simulink model "CSE1_DP"  (R2014a)
settings: Solver=ode4  StartTime=0.0  StopTime=time  FixedStep=h  RelTol=1e-3
values from neighbouring files (symbols this model uses):
  head_pitch = 0    [run_file.m]
  Head_roll = 0    [run_file.m]
  head_yaw = 0    [run_file.m]
  K_2_psi = 30    [run_file.m]
  K_2_x = 30    [run_file.m]
  K_2_y = 30    [run_file.m]
  K_3_psi = 2    [run_file.m]
  K_3_x = 2    [run_file.m]
  K_3_y = 2    [run_file.m]
  K_4_psi = 2    [run_file.m]
  K_4_x = 2    [run_file.m]
  K_4_y = 2    [run_file.m]
  K_d_psi = 8    [run_file.m]
  K_d_x = 8    [run_file.m]
  K_d_y = 8    [run_file.m]
  K_ff_r = 0    [run_file.m]
  K_ff_r_dot = 0    [run_file.m]
  K_ff_u = 0    [run_file.m]
  K_ff_u_dot = 0    [run_file.m]
  K_ff_v = 0    [run_file.m]
  K_ff_v_dot = 0    [run_file.m]
  K_i_psi = 0    [run_file.m]
  K_i_x = 0    [run_file.m]
  K_i_y = 0    [run_file.m]
  K_p_psi = 3    [run_file.m]
  K_p_x = 3    [run_file.m]
  K_p_y = 3    [run_file.m]
  K_r = 0.5    [run_file.m]
  K_u = 1    [run_file.m]
  K_v = 0.5    [run_file.m]
  L = 1    [plot_script.m]    (also in run_file.m = diag([1 1 1]))
  M = [m_11 0    0 ... (first row only)    [run_file.m]
  psi_0 = 1    [run_file.m]
  psi_ref = ref(4,:)    [plot_script.m]    (also in run_file.m = 3.14159265359)
  v_max = [0.3 0.1 1]    [run_file.m]
  w_d_psi = 2    [run_file.m]
  w_d_psi_2 = 2    [run_file.m]
  w_d_x = 1    [run_file.m]
  w_d_x_2 = 1    [run_file.m]
  w_d_y = 1    [run_file.m]
  w_d_y_2 = 1    [run_file.m]
  x_0 = 5    [run_file.m]
  x_ref = ref(2,:)    [plot_script.m]    (also in run_file.m = 4)
  y_0 = 5    [run_file.m]
  y_ref = ref(3,:)    [plot_script.m]    (also in run_file.m = 3)
  zeta_psi = 1    [run_file.m]
  zeta_psi_2 = 1    [run_file.m]
  zeta_x = 1    [run_file.m]
  zeta_x_2 = 1    [run_file.m]
  zeta_y = 1    [run_file.m]
  zeta_y_2 = 1    [run_file.m]
libraries: marine_gnc x15, simulink x2
(part 1 of 2)
settings Model: Creator=Eirik Valle  LastModifiedBy=mclab

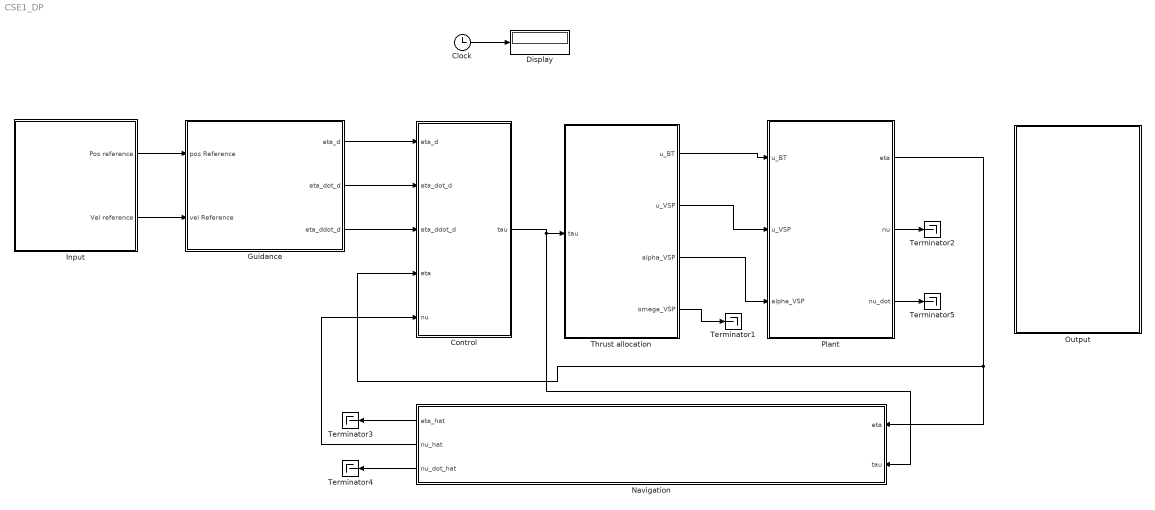
== system CSE1_DP ==
  Clock : Clock
  Control : Subsystem
  Display : Display
  Guidance : Subsystem
  Input : Subsystem
  "Navigation " : Subsystem
  Output : Subsystem
  Plant : Subsystem
  Terminator{1..5} (5 alike) : Terminator
  Thrust allocation : Subsystem
  wires:
  Control/1(tau) -> "Navigation "/2(tau), Thrust allocation/1(tau)
  Plant/1(eta) -> Control/4(eta), "Navigation "/1(eta)
  Input/1(Pos reference) -> Guidance/1("pos Reference ")
  Guidance/1(eta_d) -> Control/1(eta_d)
  Guidance/3(eta_ddot_d) -> Control/3(eta_ddot_d)
  Guidance/2(eta_dot_d) -> Control/2(eta_dot_d)
  "Navigation "/1(eta_hat) -> Terminator3/1
  "Navigation "/3(nu_dot_hat) -> Terminator4/1
  Plant/3(nu_dot) -> Terminator5/1
  Clock/1 -> Display/1
  "Navigation "/2(nu_hat) -> Control/5(nu)
  Plant/2(nu) -> Terminator2/1
  Thrust allocation/1(u_BT) -> Plant/1(u_BT)
  Thrust allocation/2(u_VSP) -> Plant/2(u_VSP)
  Thrust allocation/3(alpha_VSP) -> Plant/3(alpha_VSP)
  Thrust allocation/4(omega_VSP) -> Terminator1/1
  Input/2(Vel reference) -> Guidance/2("vel Reference ")

== system CSE1_DP/Control ==
  eta_d : Inport
  eta_dot_d : Inport  Port=2
  eta_ddot_d : Inport  Port=3
  eta : Inport  Port=4
  nu : Inport  Port=5
  Adaptive law : Subsystem  Commented=on
  Backstepping : Subsystem  Commented=on
  DP Controller : Subsystem
  MRAC : Subsystem  Commented=on
  Manual Switch : ManualSwitch  Commented=on
  tau : Outport
  tag scope: tau=global
  wires:
  eta_d/1 -> DP Controller/1(eta_d)
  eta/1 -> DP Controller/2(eta)
  nu/1 -> DP Controller/3(nu)
  DP Controller/1(tau) -> tau/1, [tau]
  eta_ddot_d/1 -> DP Controller/5(eta_ddot)
  eta_dot_d/1 -> DP Controller/4(eta_dot_d)
  Adaptive law/1(theta) -> MRAC/7(theta)

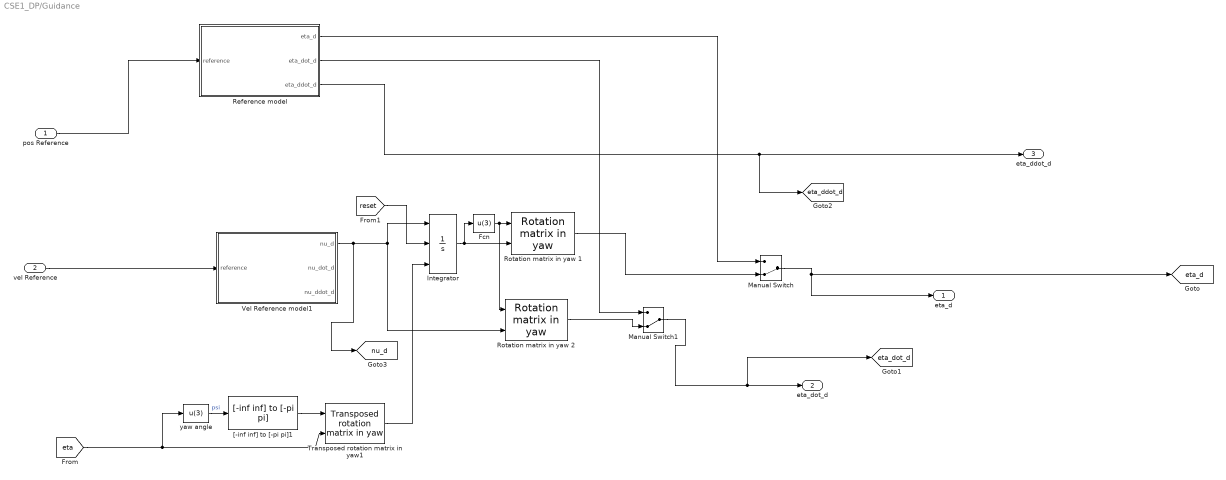
== system CSE1_DP/Guidance ==
  "pos Reference " : Inport
  "vel Reference " : Inport  Port=2
  Fcn : Fcn  Expr=u(3)
  Integrator : Integrator  ExternalReset=either  InitialConditionSource=external
  Manual Switch : ManualSwitch  CurrentSetting=0
  Manual Switch1 : ManualSwitch  CurrentSetting=0
  Reference model : Subsystem
  Rotation matrix in yaw 1 : marine_gnc/Models/ Kinematics/Rotation matrix in yaw 
  Rotation matrix in yaw 2 : marine_gnc/Models/ Kinematics/Rotation matrix in yaw 
  Transposed rotation matrix in yaw1 : marine_gnc/Models/ Kinematics/Transposed rotation  matrix in yaw
  Vel Reference model1 : Subsystem
  "[-inf inf] to [-pi pi]1" : marine_gnc/Utilities/Math Operations/[-inf inf] to [-pi pi]
  yaw angle : Fcn  Expr=u(3)
  eta_d : Outport
  eta_dot_d : Outport  Port=2
  eta_ddot_d : Outport  Port=3
  tag scope: eta_d=global, eta_ddot_d=global, eta_dot_d=global, nu_d=global
  wires:
  Manual Switch/1 -> eta_d/1, [eta_d]
  Manual Switch1/1 -> [eta_dot_d], eta_dot_d/1
  Reference model/3(eta_ddot_d) -> [eta_ddot_d], eta_ddot_d/1
  "pos Reference "/1 -> Reference model/1(reference)
  "vel Reference "/1 -> Vel Reference model1/1(reference)
  Integrator/1 -> Fcn/1, Rotation matrix in yaw 1/2
  Rotation matrix in yaw 1/1 -> Manual Switch/2
  Vel Reference model1/1(nu_d) -> [nu_d], Rotation matrix in yaw 2/2, Integrator/1
  Fcn/1 -> Rotation matrix in yaw 2/1, Rotation matrix in yaw 1/1
  Reference model/1(eta_d) -> Manual Switch/1
  Rotation matrix in yaw 2/1 -> Manual Switch1/2
  Reference model/2(eta_dot_d) -> Manual Switch1/1
  Transposed rotation matrix in yaw1/1 -> Integrator/3
  [reset] -> Integrator/2
  "[-inf inf] to [-pi pi]1"/1 -> Transposed rotation matrix in yaw1/1
  yaw angle/1 -> "[-inf inf] to [-pi pi]1"/1  "psi"
  [eta] -> yaw angle/1, Transposed rotation matrix in yaw1/2

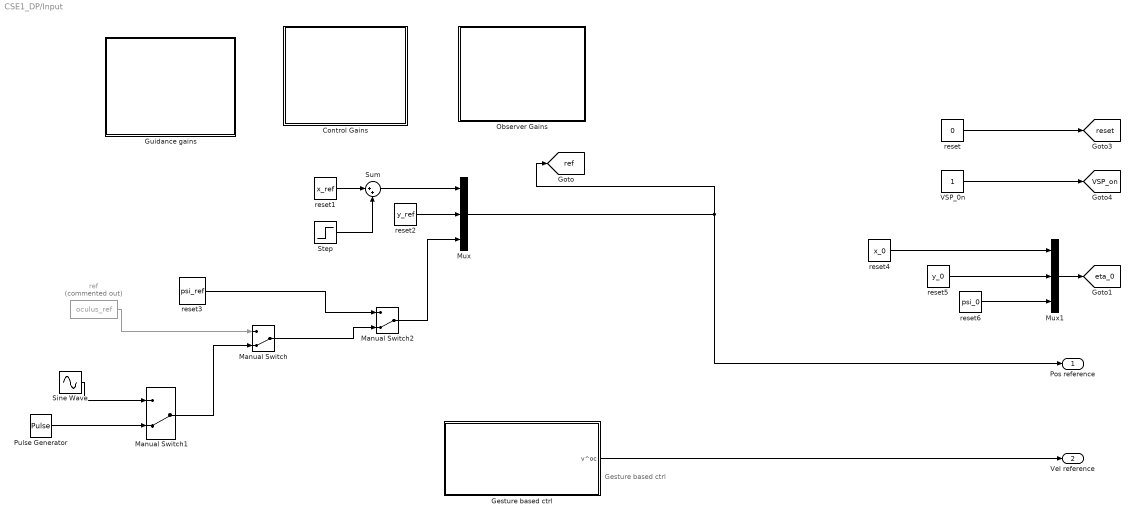
== system CSE1_DP/Input ==
  note: Gesture based ctrl
  Control Gains : Subsystem
  Gesture based ctrl : Subsystem
  Guidance gains : Subsystem
  Manual Switch : ManualSwitch  CurrentSetting=0
  Manual Switch1 : ManualSwitch  CurrentSetting=0
  Manual Switch2 : ManualSwitch  CurrentSetting=0
  Mux : Mux  Inputs=3
  Mux1 : Mux  Inputs=3
  Observer Gains : Subsystem
  Pulse Generator : DiscretePulseGenerator  PulseType=Time based  Amplitude=pi*0.9  Period=30  PulseWidth=50
  Sine Wave : Sin  Amplitude=pi/2  Frequency=0.2  SampleTime=0
  Step : Step  Time=100  After=2  SampleTime=0
  Sum : Sum  Inputs=|++
  VSP_0n : Constant
  ref : FromWorkspace  Commented=on  VariableName=oculus_ref  SampleTime=0
  reset : Constant  Value=0
  reset1 : Constant  Value=x_ref
  reset2 : Constant  Value=y_ref
  reset3 : Constant  Value=psi_ref
  reset4 : Constant  Value=x_0
  reset5 : Constant  Value=y_0
  reset6 : Constant  Value=psi_0
  Pos reference : Outport
  Vel reference : Outport  Port=2
  tag scope: VSP_on=global, eta_0=global, ref=global, reset=global
  wires:
  Mux/1 -> Pos reference/1, [ref]
  reset/1 -> [reset]
  VSP_0n/1 -> [VSP_on]
  reset1/1 -> Sum/1
  reset2/1 -> Mux/2
  reset3/1 -> Manual Switch2/1
  reset4/1 -> Mux1/1
  reset5/1 -> Mux1/2
  reset6/1 -> Mux1/3
  Mux1/1 -> [eta_0]
  ref/1 -> Manual Switch/1
  Manual Switch/1 -> Manual Switch2/2
  Pulse Generator/1 -> Manual Switch1/2
  Sine Wave/1 -> Manual Switch1/1
  Manual Switch1/1 -> Manual Switch/2
  Manual Switch2/1 -> Mux/3
  Sum/1 -> Mux/1
  Step/1 -> Sum/2
  Gesture based ctrl/1("v^oc ") -> Vel reference/1

== system CSE1_DP/Navigation  ==
  eta : Inport
  tau : Inport  Port=2
  Derivative filter : Subsystem
  Manual Switch : ManualSwitch  CurrentSetting=0
  Manual Switch1 : ManualSwitch  CurrentSetting=0
  Nonlinear Passisve Observer : Subsystem
  Terminator : Terminator
  tau_2_tau_actual : Subsystem
  eta_hat : Outport
  nu_hat : Outport  Port=2
  nu_dot_hat : Outport  Port=3
  tag scope: b_hat=global, eta_hat=global, nu_dot_hat=global, nu_hat=global
  wires:
  tau/1 -> Manual Switch/1, tau_2_tau_actual/1(tau)
  Nonlinear Passisve Observer/1(eta_hat) -> [eta_hat], eta_hat/1
  Manual Switch1/1 -> nu_hat/1, [nu_hat]
  Nonlinear Passisve Observer/4(b_hat) -> Terminator/1, [b_hat]
  Nonlinear Passisve Observer/3(nu_dot_hat) -> [nu_dot_hat], nu_dot_hat/1
  Manual Switch/1 -> Nonlinear Passisve Observer/2(tau)
  tau_2_tau_actual/1(tau_actual) -> Manual Switch/2
  eta/1 -> Derivative filter/1(eta), Nonlinear Passisve Observer/1(eta)
  Nonlinear Passisve Observer/2(nu_hat) -> Manual Switch1/1, tau_2_tau_actual/2(nu_hat)
  Derivative filter/1(nu_hat) -> Manual Switch1/2

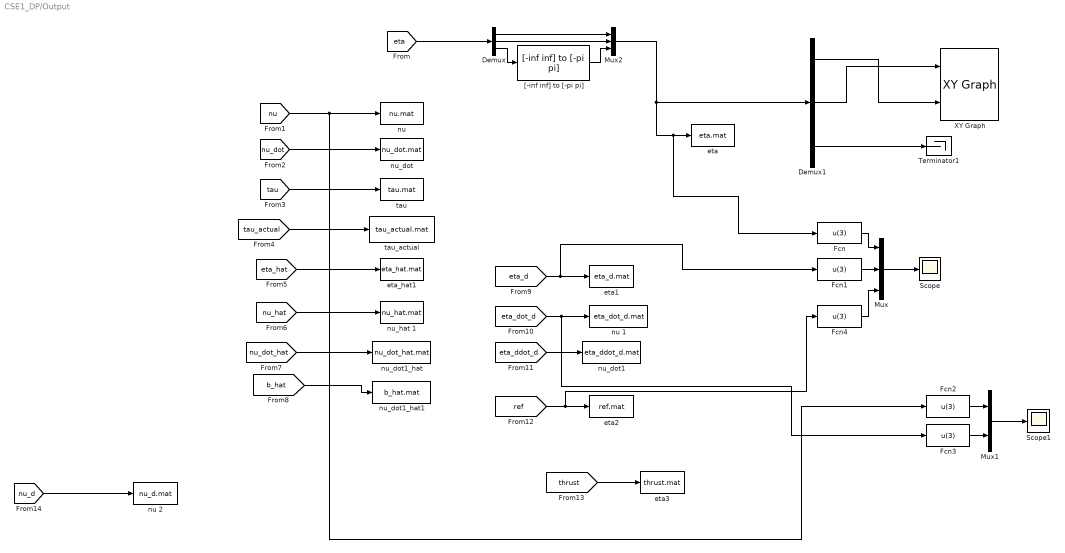
== system CSE1_DP/Output ==
  Demux : Demux  Outputs=3
  Demux1 : Demux  Outputs=3
  Fcn{,1..4} (5 alike) : Fcn  Expr=u(3)
  Mux : Mux  Inputs=3
  Mux1 : Mux  Inputs=2
  Mux2 : Mux  Inputs=3
  Scope : Scope
      settings: YMin=-3.5  YMax=3.5
  Scope1 : Scope
      settings: YMin=-0.1  YMax=0.9
  Terminator1 : Terminator
  XY Graph : simulink/Sinks/XY Graph  xmin=-10  xmax=10  ymin=-10  ymax=10  st=-1
  "[-inf inf] to [-pi pi]" : marine_gnc/Utilities/Math Operations/[-inf inf] to [-pi pi]
  eta : ToFile  Filename=eta.mat  MatrixName=eta
  eta1 : ToFile  Filename=eta_d.mat  MatrixName=eta_d
  eta2 : ToFile  Filename=ref.mat  MatrixName=ref
  eta3 : ToFile  Filename=thrust.mat  MatrixName=thrust
  eta_hat1 : ToFile  Filename=eta_hat.mat  MatrixName=eta_hat
  "nu " : ToFile  Filename=nu.mat  MatrixName=nu
  nu 1 : ToFile  Filename=eta_dot_d.mat  MatrixName=eta_dot_d
  nu 2 : ToFile  Filename=nu_d.mat  MatrixName=nu_d
  nu_dot : ToFile  Filename=nu_dot.mat  MatrixName=nu_dot
  nu_dot1 : ToFile  Filename=eta_ddot_d.mat  MatrixName=eta_ddot_d
  nu_dot1_hat : ToFile  Filename=nu_dot_hat.mat  MatrixName=nu_dot_hat
  nu_dot1_hat1 : ToFile  Filename=b_hat.mat  MatrixName=b_hat
  nu_hat 1 : ToFile  Filename=nu_hat.mat  MatrixName=nu_hat
  tau : ToFile  Filename=tau.mat  MatrixName=tau
  tau_actual : ToFile  Filename=tau_actual.mat  MatrixName=tau_actual
  wires:
  [nu] -> Fcn2/1, "nu "/1
  [nu_dot] -> nu_dot/1
  [tau] -> tau/1
  [tau_actual] -> tau_actual/1
  [eta_hat] -> eta_hat1/1
  [nu_hat] -> nu_hat 1/1
  [nu_dot_hat] -> nu_dot1_hat/1
  [b_hat] -> nu_dot1_hat1/1
  [eta_d] -> Fcn1/1, eta1/1
  [eta_ddot_d] -> nu_dot1/1
  Mux2/1 -> Fcn/1, eta/1, Demux1/1
  Demux1/3 -> Terminator1/1
  Demux1/1 -> XY Graph/2
  Demux1/2 -> XY Graph/1
  [ref] -> Fcn4/1, eta2/1
  [thrust] -> eta3/1
  Mux/1 -> Scope/1
  Fcn/1 -> Mux/1
  Fcn1/1 -> Mux/2
  [eta_dot_d] -> Fcn3/1, nu 1/1
  Mux1/1 -> Scope1/1
  Fcn2/1 -> Mux1/1
  Fcn3/1 -> Mux1/2
  Demux/1 -> Mux2/1
  Demux/2 -> Mux2/2
  "[-inf inf] to [-pi pi]"/1 -> Mux2/3
  Demux/3 -> "[-inf inf] to [-pi pi]"/1
  [eta] -> Demux/1
  Fcn4/1 -> Mux/3
  [nu_d] -> nu 2/1

== system CSE1_DP/Plant ==
  u_BT : Inport
  u_VSP : Inport  Port=2
  alpha_VSP : Inport  Port=3
  CSE1 nonlinear with thruster dynamics : Subsystem
  Terminator : Terminator
  eta : Outport
  nu : Outport  Port=2
  nu_dot : Outport  Port=3
  tag scope: eta=global, nu=global, nu_dot=global, tau_actual=global
  wires:
  CSE1 nonlinear with thruster dynamics/4(nu_dot) -> nu_dot/1, [nu_dot]
  CSE1 nonlinear with thruster dynamics/3(nu) -> [nu], nu/1
  CSE1 nonlinear with thruster dynamics/2(eta) -> eta/1, [eta]
  CSE1 nonlinear with thruster dynamics/1(tau_actual) -> [tau_actual], Terminator/1
  alpha_VSP/1 -> CSE1 nonlinear with thruster dynamics/3(alpha)
  u_VSP/1 -> CSE1 nonlinear with thruster dynamics/2(u_VSP)
  u_BT/1 -> CSE1 nonlinear with thruster dynamics/1(u_bt)

== system CSE1_DP/Thrust allocation ==
  tau : Inport
  linear thrust allocation : Subsystem
  u_BT : Outport
  u_VSP : Outport  Port=2
  alpha_VSP : Outport  Port=3
  omega_VSP : Outport  Port=4
  tag scope: thrust=global
  wires:
  tau/1 -> linear thrust allocation/1(tau)
  linear thrust allocation/5(thrust) -> [thrust]
  linear thrust allocation/1(u_BT) -> u_BT/1
  linear thrust allocation/2(u_VSP) -> u_VSP/1
  linear thrust allocation/3(alpha_VSP) -> alpha_VSP/1
  linear thrust allocation/4(omega_VSP) -> omega_VSP/1

== system CSE1_DP/Control/Adaptive law ==
  a_psi : Inport
  r : Inport  Port=2
  r_d : Inport  Port=3
  Abs : Abs
  Demux : Demux  Outputs=2
  Integrator : Integrator  InitialCondition=[0.01 0.01]
  Matrix Multiply : Product  Multiplication=Matrix(*)
  Mux2 : Mux  Inputs=2
  Product : Product
  Product2 : Product
  Sum : Sum  Inputs=|+-
  theta : Outport
  tag scope: theta_1=global, theta_2=global
  wires:
  Matrix Multiply/1 -> Integrator/1
  Product/1 -> Matrix Multiply/2
  Integrator/1 -> Demux/1, theta/1
  Sum/1 -> Product/2
  Product2/1 -> Mux2/2
  a_psi/1 -> Mux2/1
  r/1 -> Sum/1, Product2/2, Abs/1
  Abs/1 -> Product2/1
  r_d/1 -> Sum/2
  Mux2/1 -> Product/1
  Demux/1 -> [theta_1]
  Demux/2 -> [theta_2]
  [iG5] -> Matrix Multiply/1

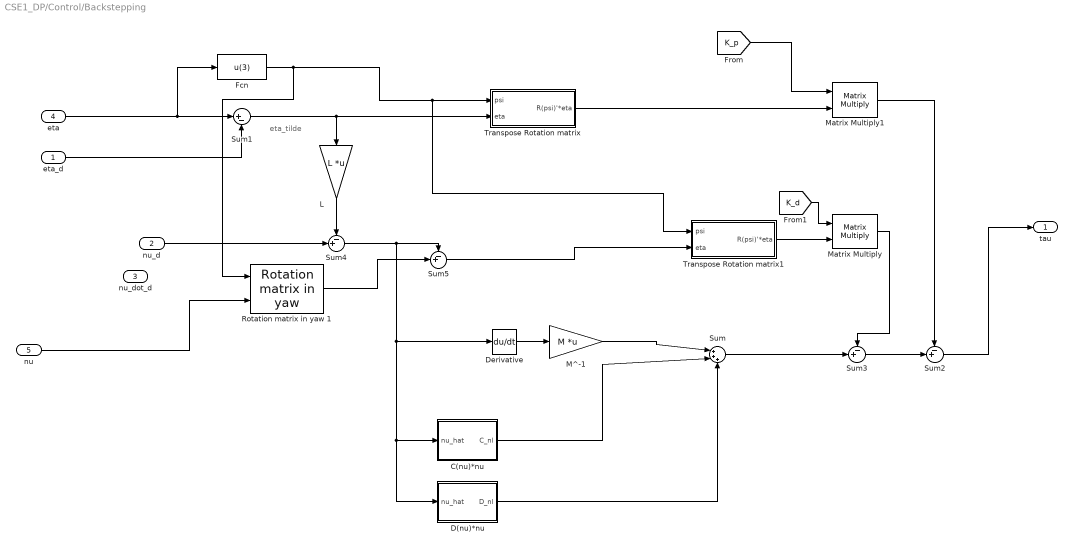
== system CSE1_DP/Control/Backstepping ==
  note: eta_tilde
  eta_d : Inport
  nu_d : Inport  Port=2
  nu_dot_d : Inport  Port=3
  eta : Inport  Port=4
  nu : Inport  Port=5
  C(nu)*nu : MATLAB Function  TreatAsAtomicUnit=on
  D(nu)*nu : MATLAB Function  TreatAsAtomicUnit=on
  Derivative : Derivative
  Fcn : Fcn  Expr=u(3)
  L : Gain  Gain=L  Multiplication=Matrix(K*u)
  M^-1 : Gain  Gain=M  Multiplication=Matrix(K*u)
  Matrix Multiply : Product  Multiplication=Matrix(*)
  Matrix Multiply1 : Product  Multiplication=Matrix(*)
  Rotation matrix in yaw 1 : marine_gnc/Models/ Kinematics/Rotation matrix in yaw 
  Sum : Sum  Inputs=|+++
  Sum1 : Sum  Inputs=|+-
  Sum{2..5} (4 alike) : Sum  Inputs=-+|
  Transpose Rotation matrix : Subsystem
  Transpose Rotation matrix1 : Subsystem
  tau : Outport
  wires:
  nu/1 -> Rotation matrix in yaw 1/2
  Derivative/1 -> M^-1/1
  M^-1/1 -> Sum/1
  C(nu)*nu/1(C_nl) -> Sum/2
  D(nu)*nu/1(D_nl) -> Sum/3
  eta/1 -> Fcn/1, Sum1/1
  eta_d/1 -> Sum1/2
  Sum1/1 -> L/1, Transpose Rotation matrix/2(eta)
  Fcn/1 -> Rotation matrix in yaw 1/1, Transpose Rotation matrix1/1(psi), Transpose Rotation matrix/1(psi)
  Sum/1 -> Sum3/2
  Transpose Rotation matrix/1(R(psi)'*eta) -> Matrix Multiply1/2
  Sum3/1 -> Sum2/2
  nu_d/1 -> Sum4/2
  L/1 -> Sum4/1
  Transpose Rotation matrix1/1(R(psi)'*eta) -> Matrix Multiply/2
  Sum5/1 -> Transpose Rotation matrix1/2(eta)
  Matrix Multiply1/1 -> Sum2/1
  [K_p] -> Matrix Multiply1/1
  [K_d] -> Matrix Multiply/1
  Matrix Multiply/1 -> Sum3/1
  Rotation matrix in yaw 1/1 -> Sum5/2
  Sum2/1 -> tau/1
  Sum4/1 -> Derivative/1, D(nu)*nu/1(nu_hat), C(nu)*nu/1(nu_hat), Sum5/1

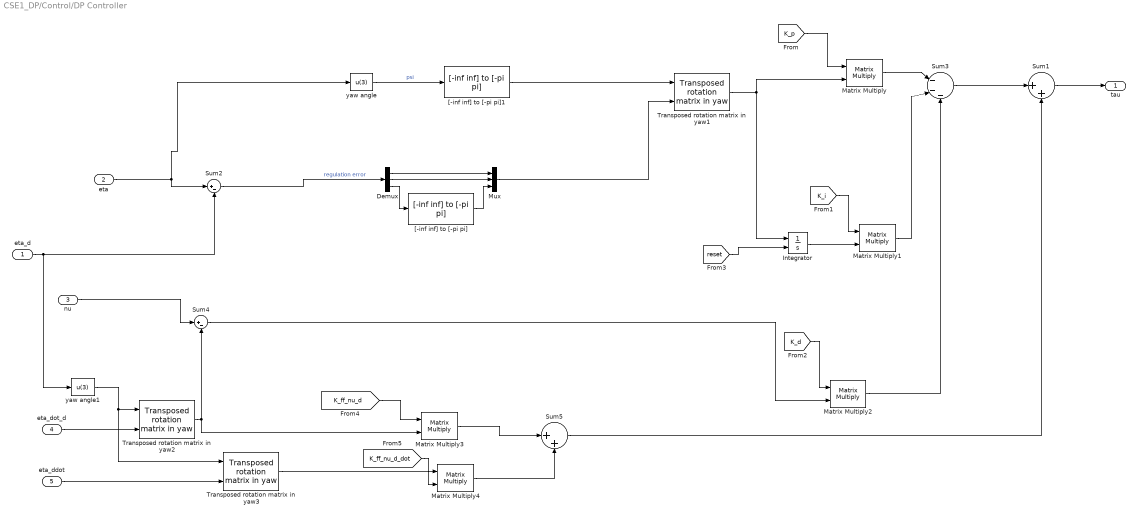
== system CSE1_DP/Control/DP Controller ==
  eta_d : Inport
  eta : Inport  Port=2
  nu : Inport  Port=3
  eta_dot_d : Inport  Port=4
  eta_ddot : Inport  Port=5
  Demux : Demux  Outputs=3
  Integrator : Integrator  ExternalReset=either
  Matrix Multiply{,1..4} (5 alike) : Product  Multiplication=Matrix(*)
  Mux : Mux  Inputs=3
  Sum1 : Sum  Inputs=|++  SaturateOnIntegerOverflow=on  InputSameDT=on  OutDataTypeStr=Inherit: Same as first input
  Sum2 : Sum  Inputs=|+-  SaturateOnIntegerOverflow=on  InputSameDT=on  OutDataTypeStr=Inherit: Same as first input
  Sum3 : Sum  Inputs=|---  SaturateOnIntegerOverflow=on  InputSameDT=on  OutDataTypeStr=Inherit: Same as first input
  Sum4 : Sum  Inputs=|+-  SaturateOnIntegerOverflow=on  InputSameDT=on  OutDataTypeStr=Inherit: Same as first input
  Sum5 : Sum  Inputs=|++  SaturateOnIntegerOverflow=on  InputSameDT=on  OutDataTypeStr=Inherit: Same as first input
  Transposed rotation matrix in yaw1 : marine_gnc/Models/ Kinematics/Transposed rotation  matrix in yaw
  Transposed rotation matrix in yaw2 : marine_gnc/Models/ Kinematics/Transposed rotation  matrix in yaw
  Transposed rotation matrix in yaw3 : marine_gnc/Models/ Kinematics/Transposed rotation  matrix in yaw
  "[-inf inf] to [-pi pi]" : marine_gnc/Utilities/Math Operations/[-inf inf] to [-pi pi]
  "[-inf inf] to [-pi pi]1" : marine_gnc/Utilities/Math Operations/[-inf inf] to [-pi pi]
  yaw angle : Fcn  Expr=u(3)
  yaw angle1 : Fcn  Expr=u(3)
  tau : Outport  InitialOutput=0
  wires:
  "[-inf inf] to [-pi pi]1"/1 -> Transposed rotation matrix in yaw1/1
  yaw angle/1 -> "[-inf inf] to [-pi pi]1"/1  "psi"
  Mux/1 -> Transposed rotation matrix in yaw1/2
  Demux/1 -> Mux/1
  Demux/2 -> Mux/2
  "[-inf inf] to [-pi pi]"/1 -> Mux/3
  Sum2/1 -> Demux/1  "regulation error"
  Demux/3 -> "[-inf inf] to [-pi pi]"/1
  Sum3/1 -> Sum1/1
  eta/1 -> Sum2/1, yaw angle/1
  nu/1 -> Sum4/1
  Matrix Multiply2/1 -> Sum3/3
  Integrator/1 -> Matrix Multiply1/2
  Matrix Multiply/1 -> Sum3/1
  Matrix Multiply1/1 -> Sum3/2
  Transposed rotation matrix in yaw1/1 -> Integrator/1, Matrix Multiply/2
  eta_d/1 -> yaw angle1/1, Sum2/2
  [reset] -> Integrator/2
  [K_p] -> Matrix Multiply/1
  [K_i] -> Matrix Multiply1/1
  [K_d] -> Matrix Multiply2/1
  eta_dot_d/1 -> Transposed rotation matrix in yaw2/2
  Transposed rotation matrix in yaw2/1 -> Sum4/2, Matrix Multiply3/2
  Sum4/1 -> Matrix Multiply2/2
  yaw angle1/1 -> Transposed rotation matrix in yaw3/1, Transposed rotation matrix in yaw2/1
  Sum1/1 -> tau/1
  eta_ddot/1 -> Transposed rotation matrix in yaw3/2
  Transposed rotation matrix in yaw3/1 -> Matrix Multiply4/2
  Matrix Multiply3/1 -> Sum5/1
  Sum5/1 -> Sum1/2
  Matrix Multiply4/1 -> Sum5/2
  [K_ff_nu_d] -> Matrix Multiply3/1
  [K_ff_nu_d_dot] -> Matrix Multiply4/1

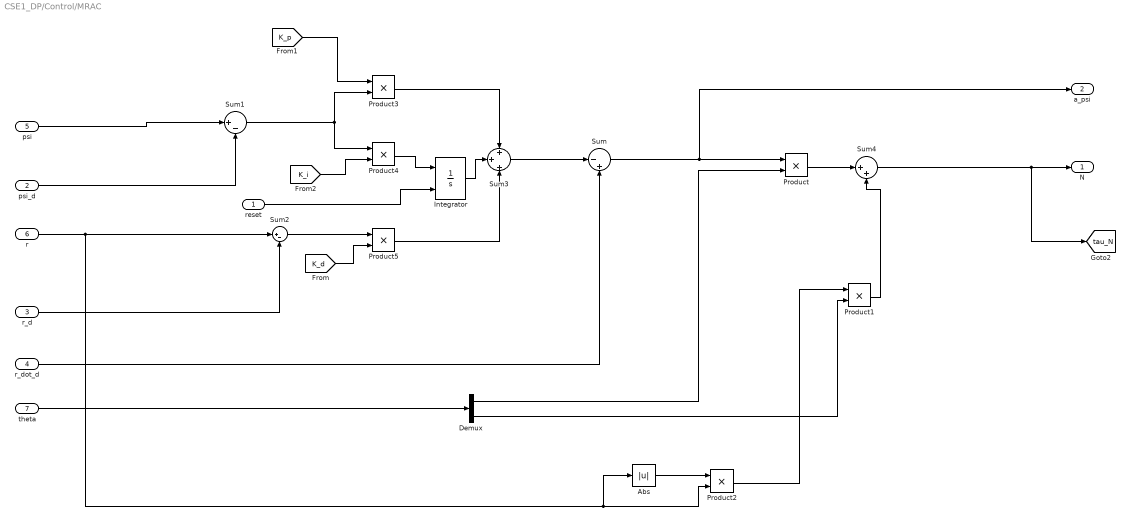
== system CSE1_DP/Control/MRAC ==
  reset : Inport
  psi_d : Inport  Port=2
  r_d : Inport  Port=3
  r_dot_d : Inport  Port=4
  psi : Inport  Port=5
  r : Inport  Port=6
  theta : Inport  Port=7
  Abs : Abs
  Demux : Demux  Outputs=2
  Integrator : Integrator  ExternalReset=either
  Product{,1..5} (6 alike) : Product
  Sum : Sum  Inputs=|-+
  Sum1 : Sum  Inputs=|+-
  Sum2 : Sum  Inputs=|+-
  Sum3 : Sum  Inputs=+|+|+
  Sum4 : Sum  Inputs=|++
  N : Outport
  a_psi : Outport  Port=2
  tag scope: tau_N=global
  wires:
  r_dot_d/1 -> Sum/2
  Sum/1 -> a_psi/1, Product/1
  psi_d/1 -> Sum1/2
  r_d/1 -> Sum2/2
  Sum2/1 -> Product5/1
  Integrator/1 -> Sum3/2
  Product5/1 -> Sum3/3
  Sum3/1 -> Sum/1
  psi/1 -> Sum1/1
  Product/1 -> Sum4/1
  r/1 -> Abs/1, Product2/2, Sum2/1
  theta/1 -> Demux/1
  Product1/1 -> Sum4/2
  Product2/1 -> Product1/1
  Abs/1 -> Product2/1
  Sum1/1 -> Product4/1, Product3/2
  Demux/1 -> Product/2
  Demux/2 -> Product1/2
  Sum4/1 -> [tau_N], N/1
  reset/1 -> Integrator/2
  Product4/1 -> Integrator/1
  [K_d] -> Product5/2
  [K_p] -> Product3/1
  Product3/1 -> Sum3/1
  [K_i] -> Product4/2

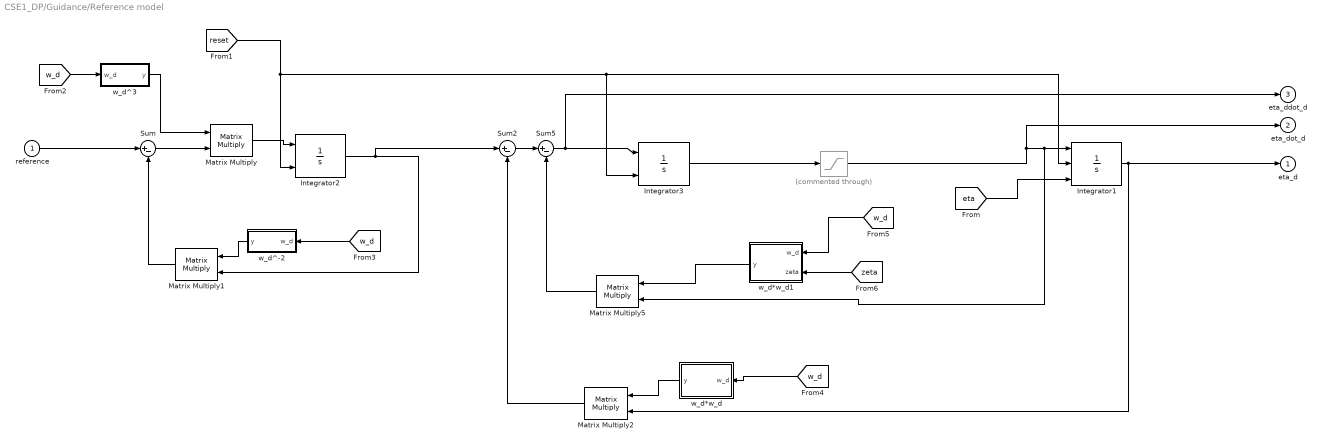
== system CSE1_DP/Guidance/Reference model ==
  reference : Inport
  "       " : Saturate  Commented=through  UpperLimit=v_max  LowerLimit=-v_max
  Integrator1 : Integrator  ExternalReset=either  InitialConditionSource=external
  Integrator2 : Integrator  ExternalReset=either
  Integrator3 : Integrator  ExternalReset=either
  Matrix Multiply{,1..2,5} (4 alike) : Product  Multiplication=Matrix(*)
  Sum : Sum  Inputs=|+-
  Sum2 : Sum  Inputs=|+-  SaturateOnIntegerOverflow=on  InputSameDT=on  OutDataTypeStr=Inherit: Same as first input
  Sum5 : Sum  Inputs=|+-  SaturateOnIntegerOverflow=on  InputSameDT=on  OutDataTypeStr=Inherit: Same as first input
  w_d*w_d : MATLAB Function  TreatAsAtomicUnit=on
  w_d*w_d1 : MATLAB Function  TreatAsAtomicUnit=on
  w_d^-2 : MATLAB Function  TreatAsAtomicUnit=on
  w_d^3 : MATLAB Function  TreatAsAtomicUnit=on
  eta_d : Outport  InitialOutput=0
  eta_dot_d : Outport  Port=2  InitialOutput=0
  eta_ddot_d : Outport  Port=3  InitialOutput=0
  wires:
  "       "/1 -> Integrator1/1, Matrix Multiply5/2, eta_dot_d/1
  Sum5/1 -> Integrator3/1, eta_ddot_d/1
  Integrator2/1 -> Sum2/1, Matrix Multiply1/2
  Sum2/1 -> Sum5/1
  Matrix Multiply2/1 -> Sum2/2
  Integrator1/1 -> eta_d/1, Matrix Multiply2/2
  Integrator3/1 -> "       "/1
  Matrix Multiply5/1 -> Sum5/2
  reference/1 -> Sum/1
  Sum/1 -> Matrix Multiply/2
  Matrix Multiply/1 -> Integrator2/1
  Matrix Multiply1/1 -> Sum/2
  [w_d] -> w_d^3/1(w_d)
  [w_d] -> w_d^-2/1(w_d)
  [w_d] -> w_d*w_d/1(w_d)
  w_d*w_d/1(y) -> Matrix Multiply2/1
  [zeta] -> w_d*w_d1/2(zeta)
  [w_d] -> w_d*w_d1/1(w_d)
  w_d*w_d1/1(y) -> Matrix Multiply5/1
  [eta] -> Integrator1/3
  [reset] -> Integrator3/2, Integrator1/2, Integrator2/2
  w_d^-2/1(y) -> Matrix Multiply1/1
  w_d^3/1(y) -> Matrix Multiply/1

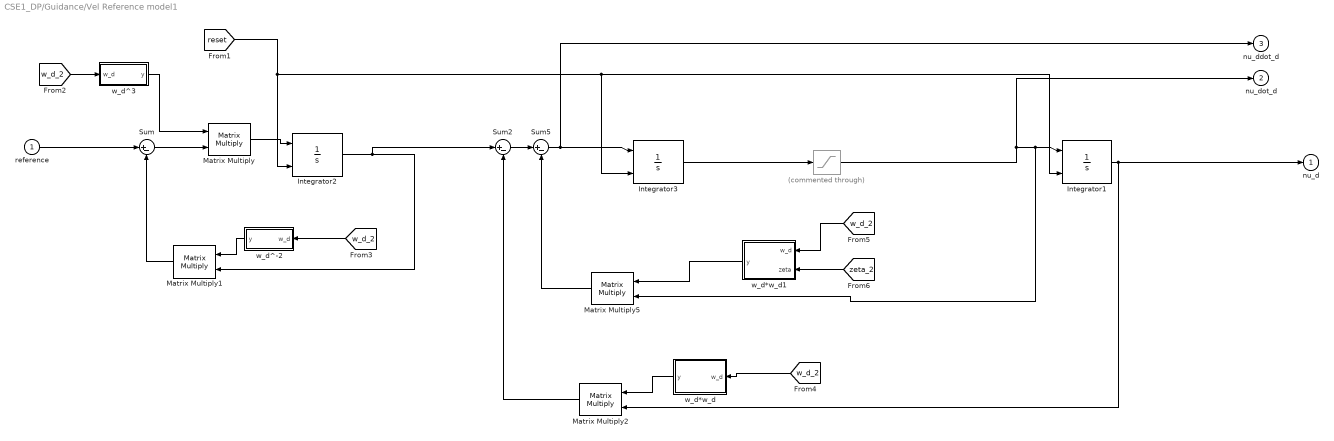
== system CSE1_DP/Guidance/Vel Reference model1 ==
  reference : Inport
  "       " : Saturate  Commented=through  UpperLimit=v_max  LowerLimit=-v_max
  Integrator1 : Integrator  ExternalReset=either
  Integrator2 : Integrator  ExternalReset=either
  Integrator3 : Integrator  ExternalReset=either
  Matrix Multiply{,1..2,5} (4 alike) : Product  Multiplication=Matrix(*)
  Sum : Sum  Inputs=|+-
  Sum2 : Sum  Inputs=|+-  SaturateOnIntegerOverflow=on  InputSameDT=on  OutDataTypeStr=Inherit: Same as first input
  Sum5 : Sum  Inputs=|+-  SaturateOnIntegerOverflow=on  InputSameDT=on  OutDataTypeStr=Inherit: Same as first input
  w_d*w_d : MATLAB Function  TreatAsAtomicUnit=on
  w_d*w_d1 : MATLAB Function  TreatAsAtomicUnit=on
  w_d^-2 : MATLAB Function  TreatAsAtomicUnit=on
  w_d^3 : MATLAB Function  TreatAsAtomicUnit=on
  nu_d : Outport  InitialOutput=0
  nu_dot_d : Outport  Port=2  InitialOutput=0
  nu_ddot_d : Outport  Port=3  InitialOutput=0
  wires:
  "       "/1 -> Integrator1/1, Matrix Multiply5/2, nu_dot_d/1
  Sum5/1 -> Integrator3/1, nu_ddot_d/1
  Integrator2/1 -> Sum2/1, Matrix Multiply1/2
  Sum2/1 -> Sum5/1
  Matrix Multiply2/1 -> Sum2/2
  Integrator1/1 -> Matrix Multiply2/2, nu_d/1
  Integrator3/1 -> "       "/1
  Matrix Multiply5/1 -> Sum5/2
  reference/1 -> Sum/1
  Sum/1 -> Matrix Multiply/2
  Matrix Multiply/1 -> Integrator2/1
  Matrix Multiply1/1 -> Sum/2
  [w_d_2] -> w_d^3/1(w_d)
  [w_d_2] -> w_d^-2/1(w_d)
  [w_d_2] -> w_d*w_d/1(w_d)
  w_d*w_d/1(y) -> Matrix Multiply2/1
  [zeta_2] -> w_d*w_d1/2(zeta)
  [w_d_2] -> w_d*w_d1/1(w_d)
  w_d*w_d1/1(y) -> Matrix Multiply5/1
  [reset] -> Integrator3/2, Integrator1/2, Integrator2/2
  w_d^-2/1(y) -> Matrix Multiply1/1
  w_d^3/1(y) -> Matrix Multiply/1

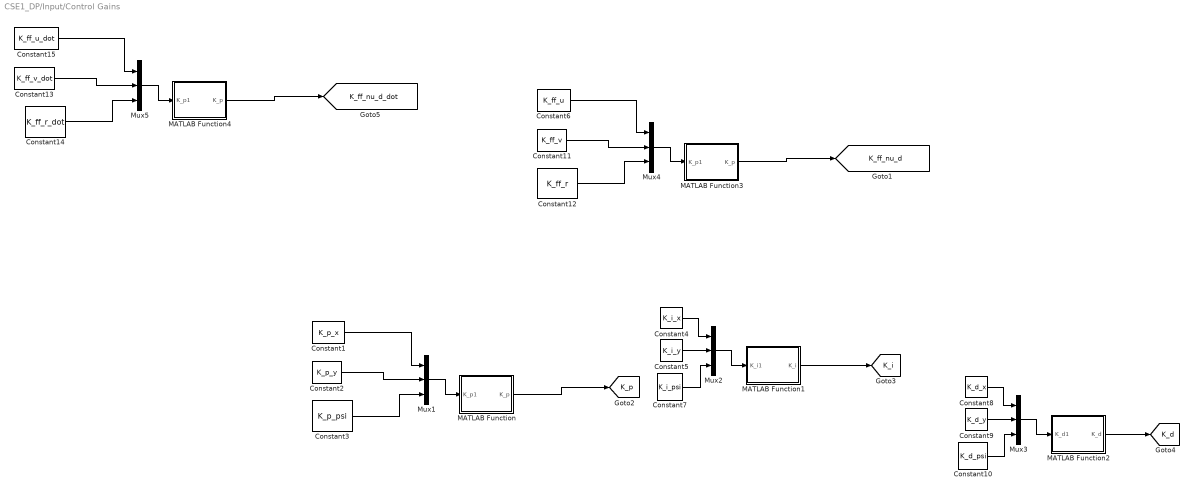
== system CSE1_DP/Input/Control Gains ==
  Constant1 : Constant  Value=K_p_x
  Constant10 : Constant  Value=K_d_psi
  Constant11 : Constant  Value=K_ff_v
  Constant12 : Constant  Value=K_ff_r
  Constant13 : Constant  Value=K_ff_v_dot
  Constant14 : Constant  Value=K_ff_r_dot
  Constant15 : Constant  Value=K_ff_u_dot
  Constant2 : Constant  Value=K_p_y
  Constant3 : Constant  Value=K_p_psi
  Constant4 : Constant  Value=K_i_x
  Constant5 : Constant  Value=K_i_y
  Constant6 : Constant  Value=K_ff_u
  Constant7 : Constant  Value=K_i_psi
  Constant8 : Constant  Value=K_d_x
  Constant9 : Constant  Value=K_d_y
  MATLAB Function : MATLAB Function  TreatAsAtomicUnit=on
  MATLAB Function1 : MATLAB Function  TreatAsAtomicUnit=on
  MATLAB Function2 : MATLAB Function  TreatAsAtomicUnit=on
  MATLAB Function3 : MATLAB Function  TreatAsAtomicUnit=on
  MATLAB Function4 : MATLAB Function  TreatAsAtomicUnit=on
  Mux{1..5} (5 alike) : Mux  Inputs=3
  tag scope: K_d=global, K_ff_nu_d=global, K_ff_nu_d_dot=global, K_i=global, K_p=global
  wires:
  Constant1/1 -> Mux1/1
  Constant3/1 -> Mux1/3
  Constant2/1 -> Mux1/2
  Mux1/1 -> MATLAB Function/1(K_p1)
  MATLAB Function/1(K_p) -> [K_p]
  Constant4/1 -> Mux2/1
  Constant7/1 -> Mux2/3
  Constant5/1 -> Mux2/2
  Mux2/1 -> MATLAB Function1/1(K_i1)
  Constant8/1 -> Mux3/1
  Constant10/1 -> Mux3/3
  Constant9/1 -> Mux3/2
  Mux3/1 -> MATLAB Function2/1(K_d1)
  MATLAB Function1/1(K_i) -> [K_i]
  MATLAB Function2/1(K_d) -> [K_d]
  Constant6/1 -> Mux4/1
  Constant12/1 -> Mux4/3
  Constant11/1 -> Mux4/2
  Mux4/1 -> MATLAB Function3/1(K_p1)
  MATLAB Function3/1(K_p) -> [K_ff_nu_d]
  Constant15/1 -> Mux5/1
  Constant14/1 -> Mux5/3
  Constant13/1 -> Mux5/2
  Mux5/1 -> MATLAB Function4/1(K_p1)
  MATLAB Function4/1(K_p) -> [K_ff_nu_d_dot]

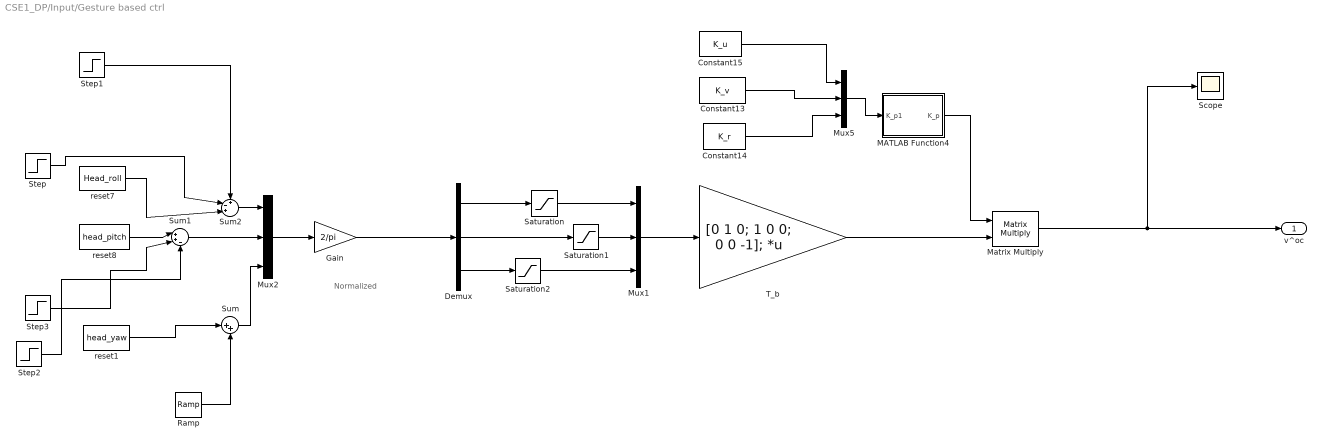
== system CSE1_DP/Input/Gesture based ctrl ==
  note: Normalized
  Constant13 : Constant  Value=K_v
  Constant14 : Constant  Value=K_r
  Constant15 : Constant  Value=K_u
  Demux : Demux  Outputs=3
  Gain : Gain  Gain=2/pi
  MATLAB Function4 : MATLAB Function  TreatAsAtomicUnit=on
  Matrix Multiply : Product  Multiplication=Matrix(*)
  Mux1 : Mux  Inputs=3
  Mux2 : Mux  Inputs=3
  Mux5 : Mux  Inputs=3
  Ramp : simulink/Sources/Ramp  slope=0.005  start=0  X0=0
  Saturation : Saturate  UpperLimit=1  LowerLimit=-1
  Saturation1 : Saturate  UpperLimit=1  LowerLimit=-1
  Saturation2 : Saturate  UpperLimit=1  LowerLimit=-1
  Scope : Scope
      settings: YMin=0  YMax=0.7  SaveName=ScopeData4
  Step : Step  Time=20  After=60*pi/180  SampleTime=0
  Step1 : Step  Time=10  After=60*pi/180  SampleTime=0
  Step2 : Step  Time=20  After=60*pi/180  SampleTime=0
  Step3 : Step  Time=10  After=60*pi/180  SampleTime=0
  Sum : Sum  Inputs=|++
  Sum1 : Sum  Inputs=|++-
  Sum2 : Sum  Inputs=+-+|
  T_b : Gain  Gain=[0 1 0; 1 0 0; 0 0 -1];  Multiplication=Matrix(K*u)
  reset1 : Constant  Value=head_yaw
  reset7 : Constant  Value=Head_roll
  reset8 : Constant  Value=head_pitch
  "v^oc " : Outport
  wires:
  reset8/1 -> Sum1/1
  reset1/1 -> Sum/1
  Mux2/1 -> Gain/1
  Gain/1 -> Demux/1
  T_b/1 -> Matrix Multiply/2
  Sum2/1 -> Mux2/1
  Sum/1 -> Mux2/3
  Sum1/1 -> Mux2/2
  Step3/1 -> Sum1/2
  reset7/1 -> Sum2/3
  Step/1 -> Sum2/2
  Step1/1 -> Sum2/1
  Step2/1 -> Sum1/3
  Ramp/1 -> Sum/2
  Demux/2 -> Saturation1/1
  Demux/1 -> Saturation/1
  Demux/3 -> Saturation2/1
  Mux1/1 -> T_b/1
  Saturation/1 -> Mux1/1
  Saturation1/1 -> Mux1/2
  Saturation2/1 -> Mux1/3
  Constant15/1 -> Mux5/1
  Constant14/1 -> Mux5/3
  Constant13/1 -> Mux5/2
  Mux5/1 -> MATLAB Function4/1(K_p1)
  MATLAB Function4/1(K_p) -> Matrix Multiply/1
  Matrix Multiply/1 -> Scope/1, "v^oc "/1

== system CSE1_DP/Input/Guidance gains ==
  Postirion guidance : Subsystem
  Velocity guidance : Subsystem

== system CSE1_DP/Input/Observer Gains ==
  Constant1 : Constant  Value=K_2_x
  Constant10 : Constant  Value=K_4_psi
  Constant2 : Constant  Value=K_2_y
  Constant3 : Constant  Value=K_2_psi
  Constant4 : Constant  Value=K_3_x
  Constant5 : Constant  Value=K_3_y
  Constant7 : Constant  Value=K_3_psi
  Constant8 : Constant  Value=K_4_x
  Constant9 : Constant  Value=K_4_y
  MATLAB Function : MATLAB Function  TreatAsAtomicUnit=on
  MATLAB Function1 : MATLAB Function  TreatAsAtomicUnit=on
  MATLAB Function2 : MATLAB Function  TreatAsAtomicUnit=on
  Mux1 : Mux  Inputs=3
  Mux2 : Mux  Inputs=3
  Mux3 : Mux  Inputs=3
  tag scope: K_2=global, K_3=global, K_4=global
  wires:
  Constant1/1 -> Mux1/1
  Constant3/1 -> Mux1/3
  Constant2/1 -> Mux1/2
  Mux1/1 -> MATLAB Function/1(K_p1)
  MATLAB Function/1(K_p) -> [K_2]
  Constant4/1 -> Mux2/1
  Constant7/1 -> Mux2/3
  Constant5/1 -> Mux2/2
  Mux2/1 -> MATLAB Function1/1(K_i1)
  Constant8/1 -> Mux3/1
  Constant10/1 -> Mux3/3
  Constant9/1 -> Mux3/2
  Mux3/1 -> MATLAB Function2/1(K_d1)
  MATLAB Function1/1(K_i) -> [K_3]
  MATLAB Function2/1(K_d) -> [K_4]

== system CSE1_DP/Navigation /Derivative filter ==
  eta : Inport
  Constant : Constant  Value=0.05
  Constant2 : Constant  Value=0.1
  Delay : Delay  DelayLength=1  InitialConditionSource=Input port  InitialCondition=0
      settings: InputPortMap=u0,p4
  Fcn : Fcn  Expr=u(3)
  Fcn1 : Fcn  Expr=u(3)
  Fcn2 : Fcn  Expr=u(3)
  MATLAB Function : MATLAB Function  TreatAsAtomicUnit=on
  MATLAB Function1 : MATLAB Function  TreatAsAtomicUnit=on
  MATLAB Function2 : MATLAB Function  TreatAsAtomicUnit=on
  MATLAB Function3 : MATLAB Function  TreatAsAtomicUnit=on
  Memory3 : Memory  X0=[0 0 0]
  Mux : Mux  Inputs=2
  Mux1 : Mux  Inputs=2
  Scope : Scope
      settings: YMin=-0.75  YMax=2  SaveName=ScopeData2
  Scope1 : Scope
      settings: YMin=-0.15  YMax=0.08  SaveName=ScopeData3
  Stepsize : Constant  Value=0.01
  nu_hat : Outport
  wires:
  eta/1 -> Fcn/1, Mux/1, MATLAB Function/2(eta)
  Fcn/1 -> MATLAB Function3/2(psi)
  Constant/1 -> MATLAB Function/1(a)
  Stepsize/1 -> MATLAB Function1/1(h)
  Memory3/1 -> MATLAB Function2/3(eta_dot_filtered_prev)
  Constant2/1 -> MATLAB Function2/1(a)
  MATLAB Function3/1(nu) -> nu_hat/1
  Mux/1 -> Scope/1
  MATLAB Function1/1(eta_dot) -> Fcn1/1, MATLAB Function2/2(eta_dot)
  MATLAB Function2/1(eta_dot_filtered) -> Fcn2/1, MATLAB Function3/1(eta_dot), Memory3/1
  Mux1/1 -> Scope1/1
  Fcn1/1 -> Mux1/1
  Fcn2/1 -> Mux1/2
  MATLAB Function/1(eta_filtered) -> Mux/2, Delay/1, MATLAB Function1/2(eta)
  Delay/1 -> MATLAB Function1/3(eta_prev), MATLAB Function/3(eta_filtered_prev)
  [eta] -> Delay/2

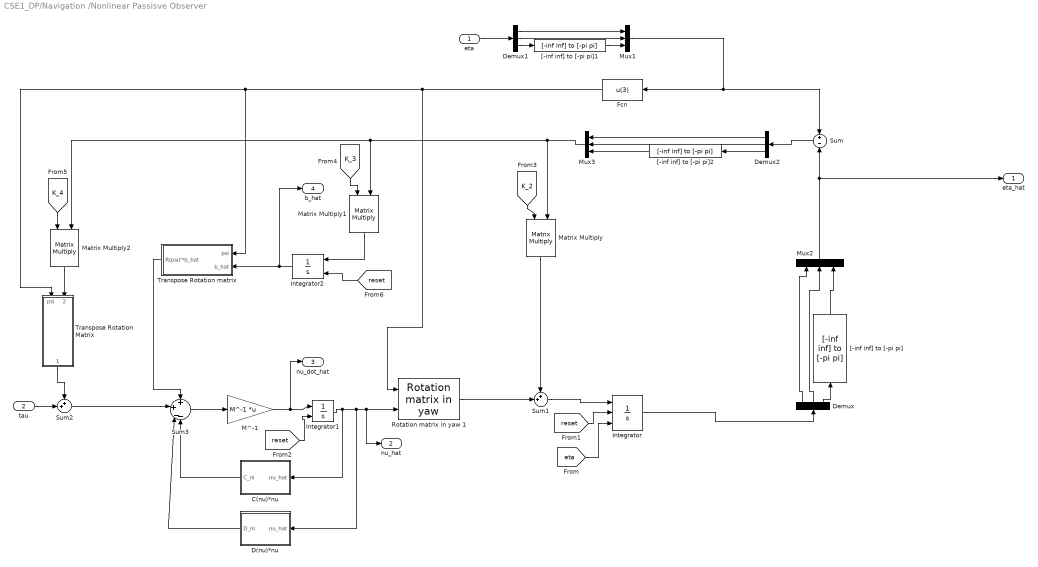
== system CSE1_DP/Navigation /Nonlinear Passisve Observer ==
  eta : Inport
  tau : Inport  Port=2
  C(nu)*nu : MATLAB Function  TreatAsAtomicUnit=on
  D(nu)*nu : MATLAB Function  TreatAsAtomicUnit=on
  Demux : Demux  Outputs=3
  Demux1 : Demux  Outputs=3
  Demux2 : Demux  Outputs=3
  Fcn : Fcn  Expr=u(3)
  Integrator : Integrator  ExternalReset=either  InitialConditionSource=external
  Integrator1 : Integrator  ExternalReset=either  InitialCondition=[0 0 0]'
  Integrator2 : Integrator  ExternalReset=either  InitialCondition=[0 0 0]'
  M^-1 : Gain  Gain=M^-1  Multiplication=Matrix(K*u)
  Matrix Multiply : Product  Multiplication=Matrix(*)
  Matrix Multiply1 : Product  Multiplication=Matrix(*)
  Matrix Multiply2 : Product  Multiplication=Matrix(*)
  Mux1 : Mux  Inputs=3
  Mux2 : Mux  Inputs=3
  Mux3 : Mux  Inputs=3
  Rotation matrix in yaw 1 : marine_gnc/Models/ Kinematics/Rotation matrix in yaw 
  Sum : Sum  Inputs=+|-
  Sum1 : Sum  Inputs=++|
  Sum2 : Sum  Inputs=++|
  Sum3 : Sum  Inputs=+|+|--
  Transpose Rotation Matrix : Subsystem
  Transpose Rotation matrix : Subsystem
  "[-inf inf] to [-pi pi]" : marine_gnc/Utilities/Math Operations/[-inf inf] to [-pi pi]
  "[-inf inf] to [-pi pi]1" : marine_gnc/Utilities/Math Operations/[-inf inf] to [-pi pi]
  "[-inf inf] to [-pi pi]2" : marine_gnc/Utilities/Math Operations/[-inf inf] to [-pi pi]
  eta_hat : Outport
  nu_hat : Outport  Port=2
  nu_dot_hat : Outport  Port=3
  b_hat : Outport  Port=4
  wires:
  Mux1/1 -> Fcn/1, Sum/1
  Sum1/1 -> Integrator/1
  Mux2/1 -> Sum/2, eta_hat/1
  Matrix Multiply/1 -> Sum1/1
  Mux3/1 -> Matrix Multiply2/2, Matrix Multiply1/2, Matrix Multiply/2
  Fcn/1 -> Rotation matrix in yaw 1/1, Transpose Rotation matrix/1(psi), Transpose Rotation Matrix/1(psi)
  tau/1 -> Sum2/2
  Matrix Multiply2/1 -> Transpose Rotation Matrix/2(y_tilde)
  Transpose Rotation Matrix/1(R(psi)'*y_tilde) -> Sum2/1
  Transpose Rotation matrix/1(R(psi)'*b_hat) -> Sum3/1
  Sum2/1 -> Sum3/2
  Sum3/1 -> M^-1/1
  M^-1/1 -> nu_dot_hat/1, Integrator1/1
  D(nu)*nu/1(D_nl) -> Sum3/3
  Integrator1/1 -> C(nu)*nu/1(nu_hat), Rotation matrix in yaw 1/2, nu_hat/1, D(nu)*nu/1(nu_hat)
  Rotation matrix in yaw 1/1 -> Sum1/2
  Integrator2/1 -> b_hat/1, Transpose Rotation matrix/2(b_hat)
  C(nu)*nu/1(C_nl) -> Sum3/4
  Demux/1 -> Mux2/1
  Demux/2 -> Mux2/2
  "[-inf inf] to [-pi pi]"/1 -> Mux2/3
  Demux/3 -> "[-inf inf] to [-pi pi]"/1
  Integrator/1 -> Demux/1
  Demux1/1 -> Mux1/1
  Demux1/2 -> Mux1/2
  "[-inf inf] to [-pi pi]1"/1 -> Mux1/3
  Demux1/3 -> "[-inf inf] to [-pi pi]1"/1
  eta/1 -> Demux1/1
  [eta] -> Integrator/3
  [reset] -> Integrator/2
  [reset] -> Integrator1/2
  [K_4] -> Matrix Multiply2/1
  [K_3] -> Matrix Multiply1/1
  [K_2] -> Matrix Multiply/1
  [reset] -> Integrator2/2
  Matrix Multiply1/1 -> Integrator2/1
  Demux2/1 -> Mux3/1
  Demux2/2 -> Mux3/2
  "[-inf inf] to [-pi pi]2"/1 -> Mux3/3
  Demux2/3 -> "[-inf inf] to [-pi pi]2"/1
  Sum/1 -> Demux2/1

== system CSE1_DP/Navigation /tau_2_tau_actual ==
  tau : Inport
  nu_hat : Inport  Port=2
  Demux : Demux  Outputs=3
  Mux2 : Mux  Inputs=3
  Terminator : Terminator
  Thrust allocation : MATLAB Function  TreatAsAtomicUnit=on
  Thruster configuration matrix : MATLAB Function  TreatAsAtomicUnit=on
  Thruster mapping : Subsystem
  tau_actual : Outport
  wires:
  Thruster configuration matrix/1(tau_u) -> Mux2/1
  Thruster configuration matrix/2(tau_v) -> Mux2/2
  Thruster configuration matrix/3(tau_r) -> Mux2/3
  Thruster mapping/1(F_y_BT) -> Thruster configuration matrix/1(F_y_BT)
  Thruster mapping/2(F_x_VSP) -> Thruster configuration matrix/2(F_x_VSP)
  Thruster mapping/3(F_y_VSP) -> Thruster configuration matrix/3(F_y_VSP)
  nu_hat/1 -> Thruster mapping/4(nu)
  Thrust allocation/1(u_BT) -> Thruster mapping/1(u_BT)
  Thrust allocation/2(u_VSP) -> Thruster mapping/2(u_VSP)
  Thrust allocation/3(alpha_VSP) -> Thruster mapping/3(alpha)
  [VSP_on] -> Thrust allocation/4(VSP_on)
  Demux/1 -> Thrust allocation/1(X)
  Demux/3 -> Thrust allocation/3(N)
  Thrust allocation/4(omega_VSP) -> Terminator/1
  Demux/2 -> Thrust allocation/2(Y)
  Mux2/1 -> tau_actual/1
  tau/1 -> Demux/1

== system CSE1_DP/Plant/CSE1 nonlinear with thruster dynamics ==
  u_bt : Inport
  u_VSP : Inport  Port=2
  alpha : Inport  Port=3
  Integrator : Integrator  ExternalReset=rising  InitialCondition=[0 0 0]'
  Integrator1 : Integrator  ExternalReset=rising  InitialConditionSource=external  InitialCondition=[0 0 0]'
  Mux2 : Mux  Inputs=3
  Thruster configuration matrix : MATLAB Function  TreatAsAtomicUnit=on
  Thruster mapping : Subsystem
  kinematics : MATLAB Function  TreatAsAtomicUnit=on
  kinetics : MATLAB Function  TreatAsAtomicUnit=on
  tau_actual : Outport
  eta : Outport  Port=2
  nu : Outport  Port=3
  nu_dot : Outport  Port=4
  wires:
  kinetics/1(nu_dot) -> nu_dot/1, Integrator/1
  kinematics/1(eta_dot) -> Integrator1/1
  [reset] -> Integrator/2, Integrator1/2
  Thruster configuration matrix/1(tau_u) -> kinetics/1(tau_u), Mux2/1
  Thruster configuration matrix/3(tau_r) -> kinetics/3(tau_r), Mux2/3
  Thruster mapping/1(F_y_BT) -> Thruster configuration matrix/1(F_y_BT)
  Thruster mapping/2(F_x_VSP) -> Thruster configuration matrix/2(F_x_VSP)
  Thruster mapping/3(F_y_VSP) -> Thruster configuration matrix/3(F_y_VSP)
  Integrator/1 -> kinematics/1(nu), nu/1, kinetics/4(nu), Thruster mapping/4(nu)
  [eta_0] -> Integrator1/3
  Integrator1/1 -> eta/1, kinematics/2(eta)
  u_bt/1 -> Thruster mapping/1(u_BT)
  u_VSP/1 -> Thruster mapping/2(u_VSP)
  alpha/1 -> Thruster mapping/3(alpha)
  Mux2/1 -> tau_actual/1
  Thruster configuration matrix/2(tau_v) -> kinetics/2(tau_v), Mux2/2

== system CSE1_DP/Thrust allocation/linear thrust allocation ==
  tau : Inport
  Demux : Demux  Outputs=3
  Mux1 : Mux  Inputs=3
  Thrust allocation : MATLAB Function  TreatAsAtomicUnit=on
  u_BT : Outport
  u_VSP : Outport  Port=2
  alpha_VSP : Outport  Port=3
  omega_VSP : Outport  Port=4
  thrust : Outport  Port=5
  wires:
  Thrust allocation/2(u_VSP) -> u_VSP/1, Mux1/1
  Thrust allocation/3(alpha_VSP) -> alpha_VSP/1, Mux1/2
  [VSP_on] -> Thrust allocation/4(VSP_on)
  Demux/1 -> Thrust allocation/1(X)
  Demux/3 -> Thrust allocation/3(N)
  Demux/2 -> Thrust allocation/2(Y)
  tau/1 -> Demux/1
  Mux1/1 -> thrust/1
  Thrust allocation/1(u_BT) -> Mux1/3, u_BT/1
  Thrust allocation/4(omega_VSP) -> omega_VSP/1

== system CSE1_DP/Control/Backstepping/Transpose Rotation matrix ==
  psi : Inport
  eta : Inport  Port=2
  Mux : Mux  Inputs=2
  Mux1 : Mux  Inputs=3
  Row1 : Fcn  Expr=cos(u(1))*u(2)+sin(u(1))*u(3)
  Row2 : Fcn  Expr=-sin(u(1))*u(2)+cos(u(1))*u(3)
  Row3 : Fcn  Expr=u(4)
  R(psi)'*eta : Outport
  wires:
  Mux/1 -> Row3/1, Row2/1, Row1/1
  Row1/1 -> Mux1/1
  Row2/1 -> Mux1/2
  Row3/1 -> Mux1/3
  Mux1/1 -> R(psi)'*eta/1
  psi/1 -> Mux/1
  eta/1 -> Mux/2

== system CSE1_DP/Control/Backstepping/Transpose Rotation matrix1 ==
  psi : Inport
  eta : Inport  Port=2
  Mux : Mux  Inputs=2
  Mux1 : Mux  Inputs=3
  Row1 : Fcn  Expr=cos(u(1))*u(2)+sin(u(1))*u(3)
  Row2 : Fcn  Expr=-sin(u(1))*u(2)+cos(u(1))*u(3)
  Row3 : Fcn  Expr=u(4)
  R(psi)'*eta : Outport
  wires:
  Mux/1 -> Row3/1, Row2/1, Row1/1
  Row1/1 -> Mux1/1
  Row2/1 -> Mux1/2
  Row3/1 -> Mux1/3
  Mux1/1 -> R(psi)'*eta/1
  psi/1 -> Mux/1
  eta/1 -> Mux/2

== system CSE1_DP/Input/Guidance gains/Postirion guidance ==
  Constant11 : Constant  Value=w_d_x
  Constant12 : Constant  Value=w_d_y
  Constant13 : Constant  Value=w_d_psi
  Constant14 : Constant  Value=zeta_x
  Constant15 : Constant  Value=zeta_y
  Constant16 : Constant  Value=zeta_psi
  Mux4 : Mux  Inputs=3
  Mux5 : Mux  Inputs=3
  diag : MATLAB Function  TreatAsAtomicUnit=on
  diag1 : MATLAB Function  TreatAsAtomicUnit=on
  tag scope: w_d=global, zeta=global
  wires:
  diag/1(w_d) -> [w_d]
  Constant11/1 -> Mux4/1
  Constant13/1 -> Mux4/3
  Constant12/1 -> Mux4/2
  Mux4/1 -> diag/1(w_d_vector)
  Constant14/1 -> Mux5/1
  Constant16/1 -> Mux5/3
  Constant15/1 -> Mux5/2
  Mux5/1 -> diag1/1(zeta_vector)
  diag1/1(Zeta) -> [zeta]

== system CSE1_DP/Input/Guidance gains/Velocity guidance ==
  Constant11 : Constant  Value=w_d_x_2
  Constant12 : Constant  Value=w_d_y_2
  Constant13 : Constant  Value=w_d_psi_2
  Constant14 : Constant  Value=zeta_x_2
  Constant15 : Constant  Value=zeta_y_2
  Constant16 : Constant  Value=zeta_psi_2
  Mux4 : Mux  Inputs=3
  Mux5 : Mux  Inputs=3
  diag : MATLAB Function  TreatAsAtomicUnit=on
  diag1 : MATLAB Function  TreatAsAtomicUnit=on
  tag scope: w_d_2=global, zeta_2=global
  wires:
  diag/1(w_d) -> [w_d_2]
  Constant11/1 -> Mux4/1
  Constant13/1 -> Mux4/3
  Constant12/1 -> Mux4/2
  Mux4/1 -> diag/1(w_d_vector)
  Constant14/1 -> Mux5/1
  Constant16/1 -> Mux5/3
  Constant15/1 -> Mux5/2
  Mux5/1 -> diag1/1(zeta_vector)
  diag1/1(Zeta) -> [zeta_2]

== system CSE1_DP/Navigation /Nonlinear Passisve Observer/Transpose Rotation Matrix ==
  psi : Inport
  y_tilde : Inport  Port=2
  Mux : Mux  Inputs=2
  Mux1 : Mux  Inputs=3
  Row1 : Fcn  Expr=cos(u(1))*u(2)+sin(u(1))*u(3)
  Row2 : Fcn  Expr=-sin(u(1))*u(2)+cos(u(1))*u(3)
  Row3 : Fcn  Expr=u(4)
  R(psi)'*y_tilde : Outport
  wires:
  Mux/1 -> Row3/1, Row2/1, Row1/1
  Row1/1 -> Mux1/1
  Row2/1 -> Mux1/2
  Row3/1 -> Mux1/3
  Mux1/1 -> R(psi)'*y_tilde/1
  psi/1 -> Mux/1
  y_tilde/1 -> Mux/2

== system CSE1_DP/Navigation /Nonlinear Passisve Observer/Transpose Rotation matrix ==
  psi : Inport
  b_hat : Inport  Port=2
  Mux : Mux  Inputs=2
  Mux1 : Mux  Inputs=3
  Row1 : Fcn  Expr=cos(u(1))*u(2)+sin(u(1))*u(3)
  Row2 : Fcn  Expr=-sin(u(1))*u(2)+cos(u(1))*u(3)
  Row3 : Fcn  Expr=u(4)
  R(psi)'*b_hat : Outport
  wires:
  Mux/1 -> Row3/1, Row2/1, Row1/1
  Row1/1 -> Mux1/1
  Row2/1 -> Mux1/2
  Row3/1 -> Mux1/3
  Mux1/1 -> R(psi)'*b_hat/1
  psi/1 -> Mux/1
  b_hat/1 -> Mux/2

== system CSE1_DP/Navigation /tau_2_tau_actual/Thruster mapping ==
  u_BT : Inport
  u_VSP : Inport  Port=2
  alpha : Inport  Port=3
  nu : Inport  Port=4
  Bow thruster : MATLAB Function  TreatAsAtomicUnit=on
  VSP : MATLAB Function  TreatAsAtomicUnit=on
  F_y_BT : Outport
  F_x_VSP : Outport  Port=2
  F_y_VSP : Outport  Port=3
  wires:
  alpha/1 -> VSP/1(alpha)
  u_VSP/1 -> VSP/2(u_VST)
  nu/1 -> Bow thruster/2(nu)
  u_BT/1 -> Bow thruster/1(u_BT)
  Bow thruster/1(F_y) -> F_y_BT/1
  VSP/1(F_x) -> F_x_VSP/1
  VSP/2(F_y) -> F_y_VSP/1

== system CSE1_DP/Plant/CSE1 nonlinear with thruster dynamics/Thruster mapping ==
  u_BT : Inport
  u_VSP : Inport  Port=2
  alpha : Inport  Port=3
  nu : Inport  Port=4
  Bow thruster : MATLAB Function  TreatAsAtomicUnit=on
  VSP : MATLAB Function  TreatAsAtomicUnit=on
  F_y_BT : Outport
  F_x_VSP : Outport  Port=2
  F_y_VSP : Outport  Port=3
  wires:
  alpha/1 -> VSP/1(alpha)
  u_VSP/1 -> VSP/2(u_VST)
  nu/1 -> Bow thruster/2(nu)
  u_BT/1 -> Bow thruster/1(u_BT)
  Bow thruster/1(F_y) -> F_y_BT/1
  VSP/1(F_x) -> F_x_VSP/1
  VSP/2(F_y) -> F_y_VSP/1

== matlab function CSE1_DP/Guidance/Reference model/w_d^3 ==
  data: w_d input; y output
function y = fcn(w_d)
%#codegen

y = w_d^3;

== matlab function CSE1_DP/Guidance/Reference model/w_d^-2 ==
  data: w_d input; y output
function y = fcn(w_d)
%#codegen

y = w_d^-2;

== matlab function CSE1_DP/Guidance/Reference model/w_d*w_d ==
  data: w_d input; y output
function y = fcn(w_d)
%#codegen

y = w_d*w_d;

== matlab function CSE1_DP/Guidance/Reference model/w_d*w_d1 ==
  data: w_d input; y output; zeta input
function y = fcn(w_d,zeta)
%#codegen

y = 2*zeta*w_d;

== matlab function CSE1_DP/Plant/CSE1 nonlinear with thruster dynamics/Thruster configuration matrix ==
  data: F_y_BT input; tau_u output; F_x_VSP input; F_y_VSP input; tau_v output; tau_r output
function [tau_u, tau_v, tau_r] = fcn(F_y_BT, F_x_VSP, F_y_VSP)
%#codegen

L_VSP = -0.4575;
L_BT = 0.3875;

u = [F_x_VSP;F_y_VSP;F_y_BT];

T = [1 0 0;
     0 1 1;
     0 L_VSP L_BT];

tau = T*u; 

tau_u = tau(1);
tau_v = tau(2);
tau_r = tau(3);

== matlab function CSE1_DP/Plant/CSE1 nonlinear with thruster dynamics/Thruster mapping/Bow thruster ==
  data: u_BT input; F_y output; nu input
function F_y = fcn(u_BT,nu)
%#codegen
u = nu(1);
% Thruster characteristics
if u_BT > 0.0879
    a =       2.515;
    b =      0.1174;
    c =      -2.807;
    d =      -1.131;
    y0 = a*exp(b*u_BT) + c*exp(d*u_BT);
elseif u_BT < -0.059
    a =        -548;
    b =       0.193;
    c =       548.2;
    d =      0.1992;
    y0 = a*exp(b*u_BT) + c*exp(d*u_BT);
else
    y0 = 0;
end
% Thruster losses due to forward speed
a0 =      0.7561;
a1 =      0.3075;
b1 =      -10.22;
c1 =       2.947;
F_y = y0*(a0 + a1*atan(b1*u +c1))/1.1385;

== matlab function CSE1_DP/Plant/CSE1 nonlinear with thruster dynamics/Thruster mapping/VSP ==
  data: alpha input; F_x output; u_VST input; F_y output
function [ F_x , F_y ] = fcn(alpha,u_VST)
%#codegen
% Calculating the force in x-direction
a1 =       1.107  ;
b1 =       1.001  ;
c1 =       1.564  ;
a2 =      0.3471 ;
b2 =      0.1397 ;
c2 =      -1.599  ;
a3 =      0.1558 ;
b3 =       1.993  ;
c3 =       1.886  ;
a4 =      0.1599 ;
b4 =       0.218  ;
c4 =       1.513  ;
a5 =     0.08237 ;
b5 =       2.986  ;
c5 =      -1.601  ;
a6 =     0.04641 ;
b6 =       3.964  ;
c6 =       1.738  ;
F_x =   u_VST*( a1*sin(b1*alpha+c1) + ...
                a2*sin(b2*alpha+c2) + ...
                a3*sin(b3*alpha+c3) + ...
                a4*sin(b4*alpha+c4) + ...
                a5*sin(b5*alpha+c5) + ...
                a6*sin(b6*alpha+c6) );
% Calculating the force in y-direction
a1 =      0.7936 ;
b1 =       1.001  ;
c1 =     0.01605;
a2 =      0.2112 ;
b2 =       1.997  ;
c2 =     0.03229;
a3 =     0.07608;
b3 =       2.991  ;
c3 =       2.986  ;
a4 =     0.04817;
b4 =       3.999  ;
c4 =     -0.8668 ;
a5 =     0.01757;
b5 =       4.904  ;
c5 =      -2.622 ;
a6 =    -0.02089;
b6 =       5.068  ;
c6 =      0.2548 ;
F_y =   u_VST*( a1*sin(b1*alpha+c1) + ...
                a2*sin(b2*alpha+c2) + ...
                a3*sin(b3*alpha+c3) + ...
                a4*sin(b4*alpha+c4) + ...
                a5*sin(b5*alpha+c5) + ...
                a6*sin(b6*alpha+c6));

== matlab function CSE1_DP/Plant/CSE1 nonlinear with thruster dynamics/kinematics ==
  data: nu input; eta_dot output; eta input
function eta_dot = CSE1_eta_dot(nu,eta)

psi = eta(3);

J = [cos(psi) -sin(psi) 0
     sin(psi) cos(psi)  0
     0        0         1];

eta_dot = J*nu;

== matlab function CSE1_DP/Thrust allocation/linear thrust allocation/Thrust allocation ==
  data: X input; Y input; u_BT output; N input; u_VSP output; alpha_VSP output; VSP_on input; omega_VSP output
function [u_BT,u_VSP,alpha_VSP,omega_VSP]= fcn(X,Y,N, VSP_on)

% Forces and moments vector
tau = [X
       Y
       N];

% Extended thrust configuration matrix
l_VSP = -0.4575;
l_BT  = 0.3875;
T = [1 0     0
     0 1     1
     0 l_VSP l_BT];

% Extended thrust coefficient matrix
F_max_VSP = 1.165;
F_max_BT  = 2.629;
K = [F_max_VSP 0         0
     0         F_max_VSP 0
     0         0         F_max_BT];

% tau = T*K*u inverse
u = K\(T\tau);

u_BT      = u(3);

u_VSP_x   = u(1);
u_VSP_y   = u(2);
u_VSP     = sqrt(u_VSP_x^2 + u_VSP_y^2);
alpha_VSP = atan2(u_VSP_y,u_VSP_x);

if VSP_on
    omega_VSP = 0.3;
else
    omega_VSP = 0;
end

== matlab function CSE1_DP/Plant/CSE1 nonlinear with thruster dynamics/kinetics ==
  data: tau_u input; tau_v input; tau_r input; nu_dot output; nu input
function nu_dot = CSE1_nu_dot(tau_u,tau_v,tau_r,nu)

u   = nu(1);
v   = nu(2);
r   = nu(3);

tau = [tau_u;tau_v;tau_r];
%% MATRICES

m    = 14.79;   I_z  =  1.7600;   x_g = 0.0375;       % x_g  =  0.0460; % Table B.1


%% Added mass
X_ud  =     -2.0;											% Table B.1
					Y_vd =     -10.0;	N_vd =    -0.0;		% Table B.1
					Y_rd =      -0.0;	N_rd =    -1.0;		% Table B.1

%% Total mass matrix
m_11 = m-X_ud;
m_22 = m-Y_vd;
m_23 = m*x_g-Y_rd;
m_32 = m*x_g-N_vd;
m_33 = I_z-N_rd;

M    = [m_11 0    0
        0    m_22 m_23
        0    m_32 m_33];
	
%% Damping coefficients
% Comments at the end of the lines indicate the old values used.
X_u		= -0.6555;		X_v		= 0;
X_uu 	= 0.3545;		X_vv	= -2.443;
X_uuu 	= -3.787;		X_vvv	= 0;

						Y_v		= -1.33; 			Y_r		= -7.250; % Y_r
						Y_vv	= -2.776;			Y_rr	= -3.450; % Y_rr
						Y_vvv	= -64.91;			Y_rrr	= 0;
						
						Y_rv	= -0.805;			Y_vr	= -0.845; % Y_rv, Y_vr

						N_v		= 0;				N_r		= -1.900; % N_r
						N_vv	= -0.2088;			N_rr	= -0.750; % N_rr
						N_vvv	= 0;				N_rrr	= 0;
						
						N_rv	= 0.130;			N_vr	= 0.080; % N_rv, N_vr

%% Correolis matrix
c_13 = -(m-Y_vd)*v-(m*x_g-Y_rd)*r;
c_23 = (m-X_ud)*u;
C    = [0     0     c_13
        0     0     c_23
        -c_13 -c_23 0   ];

%% Assembly of the damping matrix
d_11 = -X_u - X_uu*u - X_uuu*u^2;
d_22 = -Y_v - Y_vv*v - Y_vvv*v^2 - Y_rv*abs(r);
d_33 = -N_r - N_rr*abs(r) - N_rrr*r^2 - N_vr*abs(v); % using abs(r)

d_12 = -X_v - X_vv*v - X_vvv*v^2;
d_23 = -Y_r - Y_rr*abs(r) - Y_rrr*r^2 - Y_vr*abs(v);
d_32 = -N_v - N_vv*v - N_vvv*v^2 - N_rv*abs(r);

D    = [d_11 d_12 0
        0    d_22 d_23
        0    d_32 d_33];



%% CALCULATION
nu_dot = M\(tau-(C+D)*nu);

== matlab function CSE1_DP/Navigation /tau_2_tau_actual/Thrust allocation ==
  data: X input; Y input; u_BT output; N input; u_VSP output; alpha_VSP output; VSP_on input; omega_VSP output
function [u_BT,u_VSP,alpha_VSP,omega_VSP]= fcn(X,Y,N, VSP_on)

% Forces and moments vector
tau = [X
       Y
       N];

% Extended thrust configuration matrix
l_VSP = -0.4575;
l_BT  = 0.3875;
T = [1 0     0
     0 1     1
     0 l_VSP l_BT];

% Extended thrust coefficient matrix
F_max_VSP = 1.165;
F_max_BT  = 2.629;
K = [F_max_VSP 0         0
     0         F_max_VSP 0
     0         0         F_max_BT];

% tau = T*K*u inverse
u = (T*K)\tau;

u_BT      = u(3);

u_VSP_x   = u(1);
u_VSP_y   = u(2);
u_VSP     = sqrt(u_VSP_x^2 + u_VSP_y^2);
alpha_VSP = atan2(u_VSP_y,u_VSP_x);

if VSP_on
    omega_VSP = 0.3;
else
    omega_VSP = 0;
end

== matlab function CSE1_DP/Navigation /tau_2_tau_actual/Thruster configuration matrix ==
  data: F_y_BT input; tau_u output; F_x_VSP input; F_y_VSP input; tau_v output; tau_r output
function [tau_u, tau_v, tau_r] = fcn(F_y_BT, F_x_VSP, F_y_VSP)
%#codegen

L_VSP = -0.4575;
L_BT = 0.3875;

u = [F_x_VSP;F_y_VSP;F_y_BT];

T = [1 0 0;
     0 1 1;
     0 L_VSP L_BT];

tau = T*u; 

tau_u = tau(1);
tau_v = tau(2);
tau_r = tau(3);

== matlab function CSE1_DP/Navigation /tau_2_tau_actual/Thruster mapping/Bow thruster ==
  data: u_BT input; F_y output; nu input
function F_y = fcn(u_BT,nu)
%#codegen
u = nu(1);
% Thruster characteristics
if u_BT > 0.0879
    a =       2.515;
    b =      0.1174;
    c =      -2.807;
    d =      -1.131;
    y0 = a*exp(b*u_BT) + c*exp(d*u_BT);
elseif u_BT < -0.059
    a =        -548;
    b =       0.193;
    c =       548.2;
    d =      0.1992;
    y0 = a*exp(b*u_BT) + c*exp(d*u_BT);
else
    y0 = 0;
end
% Thruster losses due to forward speed
a0 =      0.7561;
a1 =      0.3075;
b1 =      -10.22;
c1 =       2.947;
F_y = y0*(a0 + a1*atan(b1*u +c1))/1.1385;

== matlab function CSE1_DP/Navigation /Nonlinear Passisve Observer/D(nu)*nu ==
  data: nu_hat input; D_nl output
function D_nl = fcn(nu_hat)
%#codegen
u = nu_hat(1);
v = nu_hat(2);
r = nu_hat(3);

D_NL = D(u,v,r);

D_nl =D_NL*nu_hat;

== matlab function CSE1_DP/Navigation /Nonlinear Passisve Observer/C(nu)*nu ==
  data: nu_hat input; C_nl output
function C_nl = fcn(nu_hat)
%#codegen
u = nu_hat(1);
v = nu_hat(2);
r = nu_hat(3);

C_NL = C(u,v,r);

C_nl =C_NL*nu_hat;

== matlab function CSE1_DP/Input/Control Gains/MATLAB Function ==
  data: K_p output; K_p1 input
function K_p = fcn(K_p1)
%#codegen

K_p = diag(K_p1);

== matlab function CSE1_DP/Input/Control Gains/MATLAB Function1 ==
  data: K_i output; K_i1 input
function K_i = fcn(K_i1)
%#codegen

K_i = diag(K_i1);

== matlab function CSE1_DP/Input/Control Gains/MATLAB Function2 ==
  data: K_d output; K_d1 input
function K_d = fcn(K_d1)
%#codegen

K_d = diag(K_d1);

== matlab function CSE1_DP/Navigation /tau_2_tau_actual/Thruster mapping/VSP ==
  data: alpha input; F_x output; u_VST input; F_y output
function [ F_x , F_y ] = fcn(alpha,u_VST)
%#codegen
% Calculating the force in x-direction
a1 =       1.107  ;
b1 =       1.001  ;
c1 =       1.564  ;
a2 =      0.3471 ;
b2 =      0.1397 ;
c2 =      -1.599  ;
a3 =      0.1558 ;
b3 =       1.993  ;
c3 =       1.886  ;
a4 =      0.1599 ;
b4 =       0.218  ;
c4 =       1.513  ;
a5 =     0.08237 ;
b5 =       2.986  ;
c5 =      -1.601  ;
a6 =     0.04641 ;
b6 =       3.964  ;
c6 =       1.738  ;
F_x =   u_VST*( a1*sin(b1*alpha+c1) + ...
                a2*sin(b2*alpha+c2) + ...
                a3*sin(b3*alpha+c3) + ...
                a4*sin(b4*alpha+c4) + ...
                a5*sin(b5*alpha+c5) + ...
                a6*sin(b6*alpha+c6) );
% Calculating the force in y-direction
a1 =      0.7936 ;
b1 =       1.001  ;
c1 =     0.01605;
a2 =      0.2112 ;
b2 =       1.997  ;
c2 =     0.03229;
a3 =     0.07608;
b3 =       2.991  ;
c3 =       2.986  ;
a4 =     0.04817;
b4 =       3.999  ;
c4 =     -0.8668 ;
a5 =     0.01757;
b5 =       4.904  ;
c5 =      -2.622 ;
a6 =    -0.02089;
b6 =       5.068  ;
c6 =      0.2548 ;
F_y =   u_VST*( a1*sin(b1*alpha+c1) + ...
                a2*sin(b2*alpha+c2) + ...
                a3*sin(b3*alpha+c3) + ...
                a4*sin(b4*alpha+c4) + ...
                a5*sin(b5*alpha+c5) + ...
                a6*sin(b6*alpha+c6));

== matlab function CSE1_DP/Control/Backstepping/C(nu)*nu ==
  data: nu_hat input; C_nl output
function C_nl = fcn(nu_hat)
%#codegen
u = nu_hat(1);
v = nu_hat(2);
r = nu_hat(3);

C_NL = C(u,v,r);

C_nl =C_NL*nu_hat;

== matlab function CSE1_DP/Control/Backstepping/D(nu)*nu ==
  data: nu_hat input; D_nl output
function D_nl = fcn(nu_hat)
%#codegen
u = nu_hat(1);
v = nu_hat(2);
r = nu_hat(3);

D_NL = D(u,v,r);

D_nl =D_NL*nu_hat;

== matlab function CSE1_DP/Input/Observer Gains/MATLAB Function ==
  data: K_p output; K_p1 input
function K_p = fcn(K_p1)
%#codegen

K_p = diag(K_p1);

== matlab function CSE1_DP/Input/Observer Gains/MATLAB Function1 ==
  data: K_i output; K_i1 input
function K_i = fcn(K_i1)
%#codegen

K_i = diag(K_i1);
